simulink library "ammclib_bam"  (Simulink 9.3)
settings: Solver=VariableStepAuto  StartTime=0.0  StopTime=10.0  RelTol=1e-3
(part 1 of 15)
settings Model: Creator=ZCZ01vav01-svc  LastModifiedBy=ZCZ01vav01-svc

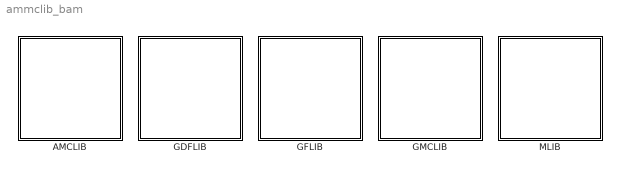
== system ammclib_bam ==
  AMCLIB : Subsystem
  GDFLIB : Subsystem
  GFLIB : Subsystem
  GMCLIB : Subsystem
  MLIB : Subsystem

== system ammclib_bam/AMCLIB ==
  F16 : Subsystem
  F32 : Subsystem

== system ammclib_bam/GDFLIB ==
  F16 : Subsystem
  F32 : Subsystem

== system ammclib_bam/GFLIB ==
  F16 : Subsystem
  F32 : Subsystem

== system ammclib_bam/GMCLIB ==
  F16 : Subsystem
  F32 : Subsystem

== system ammclib_bam/MLIB ==
  F16 : Subsystem
  F32 : Subsystem
  F32F16F16 : Subsystem
